simulink model "selectOneCh"  (R2024b)
settings: Solver=VariableStepAuto  StartTime=0.0  StopTime=5  RelTol=1e-3
model workspace (MAT data in the model file):
  sample = 1024
libraries: dspsnks4 x1, dspsrcs4 x1, dspmtrx3 x1
settings Model: Creator=asumo  LastModifiedBy=aclab_SK24
settings SolverCC: DateTimeAtSimulationTimeZero=[]

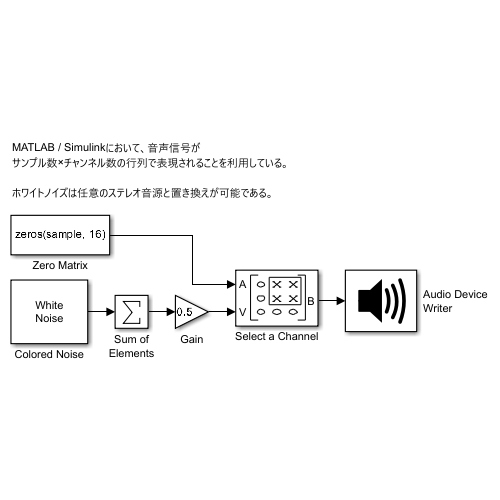
[thumbnail: Simulink's stored preview of the top-level diagram]
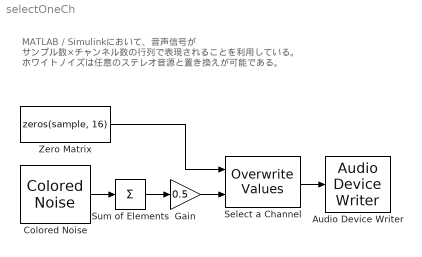
== system selectOneCh ==
  note: MATLAB / Simulinkにおいて、音声信号が
      | サンプル数×チャンネル数の行列で表現されることを利用している。
      |
      | ホワイトノイズは任意のステレオ音源と置き換えが可能である。
  Audio Device Writer : dspsnks4/Audio Device Writer  Driver=ASIO  Device=Dante Virtual Soundcard (x64)  InheritSampleRate=on  SampleRate=44100  BitDepth=32-bit float  BufferSize=4096  NumBuffers=10  DefaultOutputChannelMapping=on  OutputChannelMapping=1:2  OutputNumUnderrunSamples=off  DriverIdx=3  DeviceWarnFlag=''
  Colored Noise : dspsrcs4/Colored Noise  Color=white  InverseFrequencyPower=1  BoundedOutput=on  NumChannels=2  OutputDataType=double  SamplesPerFrame=1024  SampleTime=1  RandomStream=mt19937ar with seed  Seed=67  SimulateUsing=Interpreted execution
      settings: LibrarySourceBlock=audiosources/Colored Noise
  Gain : Gain  Gain=0.5
  Select a Channel : dspmtrx3/Overwrite Values  OverWriteDiag=Submatrix  valFrom2ndIP=Second input port  ConstValue=0  RowSpan=All rows  RowStartMode=First  RowStartIndex=1  RowEndMode=Last  RowEndIndex=1  ColSpan=One column  ColStartMode=Index  ColStartIndex=6  ColEndMode=Last  ColEndIndex=1  DiagSpan=Range of elements  DiagStartMode=Index  DiagStartIndex=2  DiagEndMode=Index  DiagEndIndex=4
  Sum of Elements : Sum  Inputs=+  CollapseMode=Specified dimension  CollapseDim=2
  Zero Matrix : Constant  Value=zeros(sample, 16)  OutDataTypeStr=double
  wires:
  Zero Matrix/1 -> Select a Channel/1
  Sum of Elements/1 -> Gain/1
  Gain/1 -> Select a Channel/2
  Colored Noise/1 -> Sum of Elements/1
  Select a Channel/1 -> Audio Device Writer/1
